simulink model "Three_Phase_Full_Wave_Rectifier_Model"  (R2020a)
settings: Solver=VariableStepAuto  StartTime=0.0  StopTime=1/60  RelTol=1e-3
libraries: powerlib x13
settings Model: Creator=Ricardo Romero  LastModifiedBy=Ricardo Romero

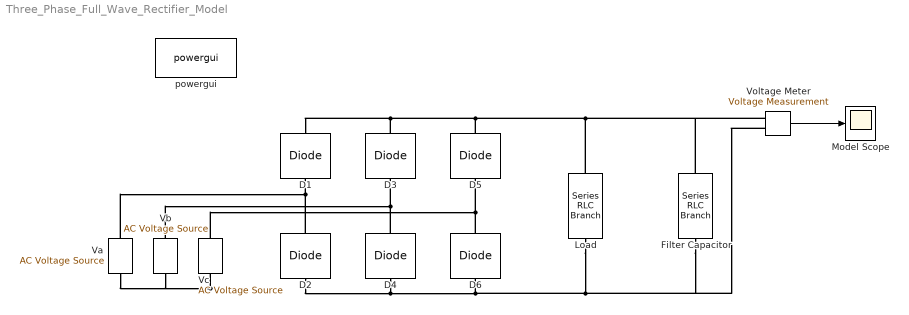
== system Three_Phase_Full_Wave_Rectifier_Model ==
  D{1..6} (6 alike) : powerlib/Power Electronics/Diode  Ron=0.001  Lon=0  Vf=0.8  IC=0  UseSnubber=0  Rs=500  Cs=250e-9  Measurements=off
  Filter Capacitor : powerlib/Elements/Series RLC Branch  LConnTagsString=__new0  RConnTagsString=__new0  BranchType=C  Resistance=10  Inductance=1e-3  SetiL0=off  InitialCurrent=0  Capacitance=1e-3  Setx0=off  InitialVoltage=0  Measurements=None
  Load : powerlib/Elements/Series RLC Branch  LConnTagsString=__new0  RConnTagsString=__new0  BranchType=R  Resistance=10  Inductance=1e-3  SetiL0=off  InitialCurrent=0  Capacitance=1e-6  Setx0=off  InitialVoltage=0  Measurements=None
  Model Scope : Scope
  Va : powerlib/Electrical Sources/AC Voltage Source  Amplitude=169.71  Phase=0  Frequency=60  SampleTime=0  Measurements=None  BusType=swing  Pref=10e3  Qref=0  Qmin=-inf  Qmax=+inf
  Vb : powerlib/Electrical Sources/AC Voltage Source  Amplitude=169.71  Phase=-120  Frequency=60  SampleTime=0  Measurements=None  BusType=swing  Pref=10e3  Qref=0  Qmin=-inf  Qmax=+inf
  Vc : powerlib/Electrical Sources/AC Voltage Source  Amplitude=169.71  Phase=120  Frequency=60  SampleTime=0  Measurements=None  BusType=swing  Pref=10e3  Qref=0  Qmin=-inf  Qmax=+inf
  Voltage Meter : powerlib/Measurements/Voltage Measurement  PhasorSimulation=off  OutputType=Complex  PSBequivalent=0
  powergui : powerlib/powergui  Priority=1  SimulationMode=Discrete  SampleTime=5e-6  frequency=60  Iterations=50  frequencyindice=60  Pbase=100e6  ErrMax=1e-4  UnitsV=kV  UnitsW=MW  buscounter=0  FunctionMessages=off  echomessages=off  EnableUseOfTLC=off  CurrentSourceSwitches=off  DisableSnubberDevices=off  DisableRonSwitches=off  DisableVfSwitches=off  DisplayEquations=off  AutomaticDiscreteSolvers=off  SolverType=Tustin/Backward Euler (TBE)  Interpol=off  ExternalGateDelay=off  methode=off  Ts=100  x0status=blocks  SPID=on  SwTol=0  HookPort=off  NonlinearTolerance=1e-4  nMaxIteration=100  ContinueOnMaxIteration=off  RestoreLinks=warning  ResistiveCurrentMeasurement=off  Frange=[0:2:500]  Ylog=off  Xlog=on  ShowGrid=off  save=off  variable=ZData  structure=0  ZoomFFT=off  StartTime=0.0  cycles=1  DisplayStyle=1  fundamental=60  FreqAxis=off  MaxFrequency=1000  frequencyindicesteady=1  RmsSteady=1  display=off
  wires:
  Voltage Meter/1 -> Model Scope/1
  connections:
  Vc/LConn1 -- Va/LConn1 -- Vb/LConn1
  D2/LConn1 -- D4/LConn1 -- Filter Capacitor/RConn1 -- Voltage Meter/LConn2 -- Load/RConn1 -- D6/LConn1
  D5/RConn1 -- Filter Capacitor/LConn1 -- Voltage Meter/LConn1 -- Load/LConn1 -- D3/RConn1 -- D1/RConn1
  D4/RConn1 -- D3/LConn1 -- Vb/RConn1
  D2/RConn1 -- Va/RConn1 -- D1/LConn1
  D6/RConn1 -- Vc/RConn1 -- D5/LConn1
